simulink model "AOC"  (R2024a)
settings: Solver=VariableStepAuto  StartTime=0.0  StopTime=600  MaxStep=1e-3  RelTol=1e-9  AbsTol=1e-10
settings Model: Creator=evgenijkondratev  LastModifiedBy=evgenijkondratev

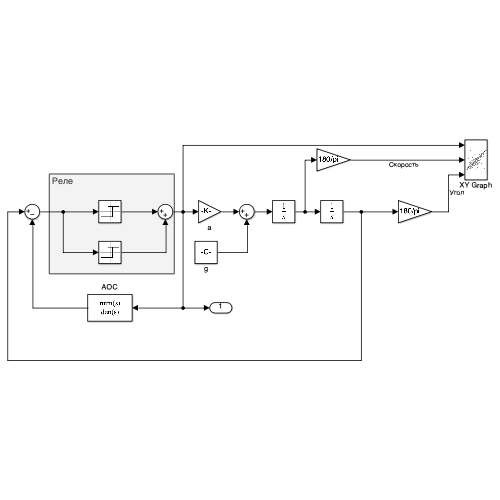
[thumbnail: Simulink's stored preview of the top-level diagram]
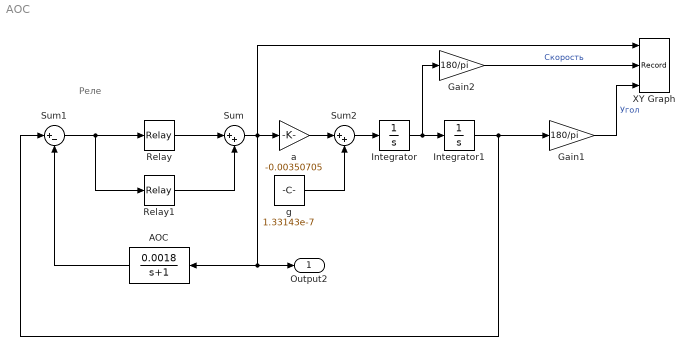
== system AOC ==
  note: Реле
  AOC : TransferFcn  Numerator=[0.0018]  Denominator=[1 1]
  Gain1 : Gain  Gain=180/pi
  Gain2 : Gain  Gain=180/pi
  Integrator : Integrator  InitialCondition=0.00048093
  Integrator1 : Integrator  InitialCondition=0.0017593
  Relay : Relay  OnSwitchValue=0.0017593  OffSwitchValue=0.0017593-0.000351870594507
  Relay1 : Relay  OnSwitchValue=-0.0017593 + 0.000351870594507  OffSwitchValue=-0.0017593  OnOutputValue=0  OffOutputValue=-1
  Sum : Sum  Inputs=|++
  Sum1 : Sum  Inputs=|+-
  Sum2 : Sum  Inputs=|++
  XY Graph : Record  FileSettingsInternal="{\"entries\":[{\"content\":{\"excelSettings\":{\"content\":{},\"type\":\"Streamout.ExcelSettings\"}},\"type\":\"Streamout.FileSettingStorage\",\"uuid\":\"\"}],\"packageUris\":[\"http:\\/\\/schema.mathworks.com\\/mf0\\/streamout_blocks\\/R2020a\"],\"version\":\"1.0\"}"  Layout=[1 1]  SignalsInternal="{\"entries\":[{\"content\":{\"signals\":[{\"content\":{\"blockPath\":[],\"dimensions\":[1],\"domain\":\"\",\"lineColor\":\"#a2142f\",\"plots\":[ 1 ],\"port\":1,\"sid\":[\"\"],\"signalID\":1,\"signalName\":\"Sum\"},\"type\":\"RecordBlkView.Signal\",\"uuid\":\"\"},{\"content\":{\"blockPath\":[],\"dimensions\":[1],\"domain\":\"\",\"lineColor\":\"#0072bd\",\"lineWidth\":20,\"plots\":[ 1 ],\"port\":2,\"sid\":[\"\"],\"signalID\":2,\"signalName\":\"Скорость\"},\"type\":\"RecordBlkView.Signal\",\"uuid\":\"\"},{\"content\":{\"blockPath\":[],\"dimensions\":[1],\"domain\":\"\",\"lineColor\":\"#fe330a\",\"lineWidth\":20,\"port\":3,\"sid\":[\"\"],\"signalID\":3,\"signalName\":\"Угол\"},\"type\":\"RecordBlkView.Signal\",\"uuid\":\"\"}]},\"type\":\"RecordBlkView.InputSignals\",\"uuid\":\"\"}],\"packageUris\":[\"http:\\/\\/schema.mathworks.com\\/mf0\\/streamout_blocks\\/R2020a\"],\"version\":\"1.0\"}"  VisualizationBindings="{\"xyplotplugin\":{\"info\":[{\"series\":[{\"bindingParametersList\":[{\"parameter\":\"X-Axis\",\"signalID\":1,\"signalName\":\"Sum\"},{\"parameter\":\"Y-Axis\",\"signalID\":2,\"signalName\":\"Скорость\"}],\"seriesID\":0}],\"subplotID\":1}]}}"  CompatibilityTag=XY
  a : Gain  Gain=-0.00350705
  g : Constant  Value=1.33143e-7
  Output2 : Outport
  wires:
  Relay/1 -> Sum/1
  Relay1/1 -> Sum/2
  Sum1/1 -> Relay/1, Relay1/1
  Sum/1 -> Output2/1, AOC/1, a/1, XY Graph/1
  Integrator/1 -> Gain2/1, Integrator1/1
  Integrator1/1 -> Sum1/1, Gain1/1
  Gain1/1 -> XY Graph/3  "Угол"
  Gain2/1 -> XY Graph/2  "Скорость"
  a/1 -> Sum2/1
  Sum2/1 -> Integrator/1
  g/1 -> Sum2/2
  AOC/1 -> Sum1/2
